simulink library "rtai_lib"  (Simulink 5.0)
settings Model: Creator=furlan  LastModifiedBy=bucher  ExtModeAutoUpdateStatusClock=off

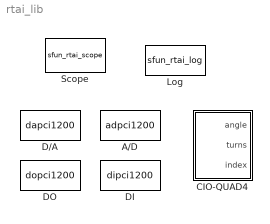
== system rtai_lib ==
  A/D : S-Function  FunctionName=adpci1200  Parameters=n_ch,ts  mask(A/D){n_ch=1, ts=0.001}
      mask prompts: n_ch "Input channels:"; ts "Sampling Time:"
      mask StyleString: popup(1|2|3|4|5|6|7|8|9|10|11|12|13|14|15|16),edit
  CIO-QUAD4 : Subsystem  mask(CIO-QUAD4){bAdd='0x300', module=1, res=1024, mode=SINGLE, counter=FIRST ONLY, rot=CLOCK, ts=0.001}
      mask prompts: bAdd "Base Address:"; res "Resolution:"; counter "Counter reset:"; rot "Rotation:"; ts "Sampling Time:"
      mask init:
      | baseAddr=hex2dec(bAdd(3:end));
      mask StyleString: edit,popup(1|2|3|4),edit,popup(SINGLE|DOUBLE|QUADRUPLE),popup(FIRST ONLY|CONTINOUS),popup(CLOCK|COUNTER CLOCK),edit
  D/A : S-Function  FunctionName=dapci1200  Parameters=n_ch,ts  mask(D/A){n_ch=1, ts=0.001}
      mask prompts: n_ch "Output channels:"; ts "Sampling Time:"
      mask StyleString: popup(1|2),edit
  DI : S-Function  FunctionName=dipci1200  Parameters=n_ch,port,ts  mask(DI){n_ch=1, port=A, ts=0.001}
      mask prompts: n_ch "Input channels:"; ts "Sampling Time:"
      mask StyleString: popup(1|2|3|4|5|6|7|8),popup(A|B),edit
  DO : S-Function  FunctionName=dopci1200  Parameters=n_ch,port,ts  mask(DO){n_ch=1, port=A, ts=0.001}
      mask prompts: n_ch "Output channels:"; ts "Sampling Time:"
      mask StyleString: popup(1|2|3|4|5|6|7|8),popup(A|B),edit
  Log : S-Function  FunctionName=sfun_rtai_log  Parameters=ts  mask{ts=0.001}
      mask prompts: ts "Sampling Time:"
  Scope : S-Function  FunctionName=sfun_rtai_scope  Parameters=numch,ts  mask{numch=1, ts=0.001}
      mask prompts: numch "Channels:"; ts "Sampling Time:"
      mask StyleString: popup(1|2|3|4|5|6),edit

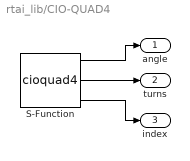
== system rtai_lib/CIO-QUAD4 ==
  S-Function : S-Function  FunctionName=cioquad4  Parameters=baseAddr,module,res,mode,counter,rot,ts
  angle : Outport
  turns : Outport  Port=2
  index : Outport  Port=3
  wires:
  S-Function/3 -> index/1
  S-Function/2 -> turns/1
  S-Function/1 -> angle/1
